simulink model "PTC_MBDS_HighpassT_RE_Sample"  (R2013a)
settings: Solver=FixedStepDiscrete  StartTime=0.0  StopTime=100  FixedStep=0.01  RelTol=1e-3
undefined symbols (not defined in the file): sigbuilder_block
libraries: simulink x2, simulink_extras x1, PTC_MBDS_LIB x1
settings Model: Creator=uidl7367  LastModifiedBy=sundeep.tuteja
settings DataIOCC: SignalLoggingSaveFormat=ModelDataLogs
settings OptimizationCC: ExpressionDepthLimit=2147483647  InitFltsAndDblsToZero=on
settings DebuggingCC: SaveWithParameterizedLinksMsg=none  SignalResolutionControl=TryResolveAllWithWarning  SolverPrmCheckMsg=none  InheritedTsInSrcMsg=none  MultiTaskDSMMsg=warning  MultiTaskCondExecSysMsg=none  FcnCallInpInsideContextMsg=UseLocalSettings  StrictBusMsg=Warning
settings RTWCC: IncludeERTFirstTime=on
settings GRTTargetCC: TargetFcnLib=ansi_tfl_tmw.mat  CombineOutputUpdateFcns=off  GRTInterface=on

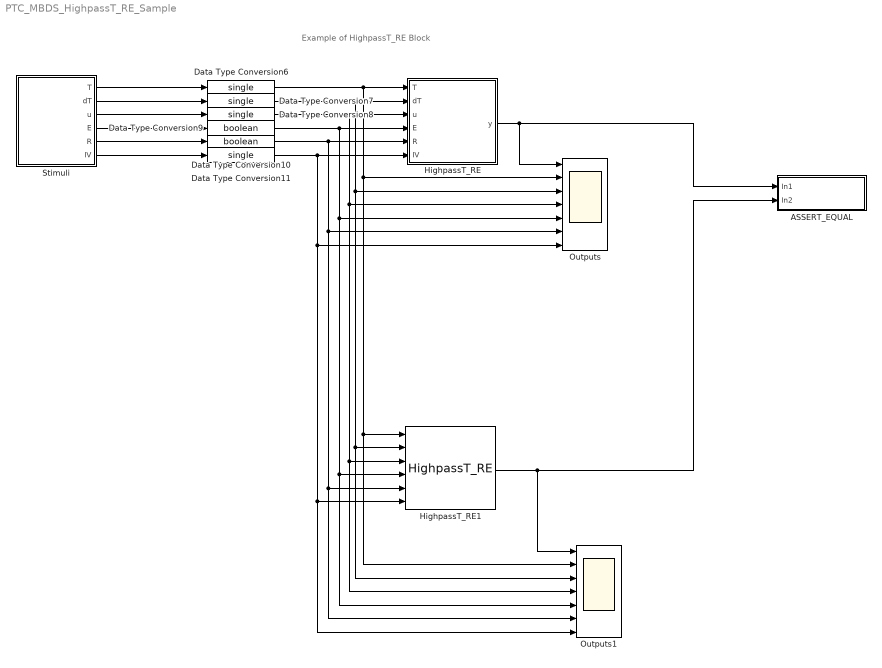
== system PTC_MBDS_HighpassT_RE_Sample ==
  note: Example of HighpassT_RE Block
  ASSERT_EQUAL : Subsystem
  Data Type Conversion10 : DataTypeConversion  InitFcn=|  OutDataTypeStr=boolean  SaturateOnIntegerOverflow=on
      | try
      |    MBDS_BlockCallback('Update', gcb);
      | end
  Data Type Conversion11 : DataTypeConversion  InitFcn=|  OutDataTypeStr=single  SaturateOnIntegerOverflow=on
      | try
      |    MBDS_BlockCallback('Update', gcb);
      | end
  Data Type Conversion6 : DataTypeConversion  InitFcn=|  OutDataTypeStr=single  SaturateOnIntegerOverflow=on
      | try
      |    MBDS_BlockCallback('Update', gcb);
      | end
  Data Type Conversion7 : DataTypeConversion  InitFcn=|  OutDataTypeStr=single  SaturateOnIntegerOverflow=on
      | try
      |    MBDS_BlockCallback('Update', gcb);
      | end
  Data Type Conversion8 : DataTypeConversion  InitFcn=|  OutDataTypeStr=single  SaturateOnIntegerOverflow=on
      | try
      |    MBDS_BlockCallback('Update', gcb);
      | end
  Data Type Conversion9 : DataTypeConversion  InitFcn=|  OutDataTypeStr=boolean  SaturateOnIntegerOverflow=on
      | try
      |    MBDS_BlockCallback('Update', gcb);
      | end
  HighpassT_RE : Subsystem  InitFcn=|  mask(HighpassT_RE){MBDS_LibraryBlock=on, dT_Enabled=on, dT=1, E_Enabled=on, R_Enabled=on, IV_Enabled=on, IV=0, MBDS_BlockVersion=05.40}
      | if(exist('MBDS_BlockCallback', 'file'))
      |    MBDS_BlockCallback('Update', gcb);
      | end
      mask prompts: MBDS_LibraryBlock "MBDS library block"; dT_Enabled "Show dT port"; dT "Sample rate (dT):"; E_Enabled "Show E port"; R_Enabled "Show R port"; IV_Enabled "Show IV port"; IV "Initial value (IV):"; MBDS_BlockVersion "Block version:"
      mask help: This block provides a discretized first order highpass filter with time constant T.
      mask init:
      | if(exist('MBDS_BlockCallback', 'file'))
      |    MBDS_BlockCallback('Init', gcb);
      | else
      |    % Disable all mask parameters
      |    MaskEnables = get_param(gcb, 'MaskEnables');
      |    for k = [1:length(MaskEnables)]
      |       MaskEnables{k} = 'off';
      |    end
      |    if(~isequal(MaskEnables, get_param(gcb, 'MaskEnables')))
      |       set_param(gcb, 'MaskEnables', MaskEnables);
      |    end
      | end
      mask Help: eval(['open([workdir(''library_dir:''),''\Blockset\help\'',get_param(gcb,''MaskType''),''.html''])'])
      mask Callback dT_Enabled:
      | % Update mask parameter dialog
      | if(exist('MBDS_BlockCallback', 'file'))
      |    MBDS_BlockCallback('dT_Enabled', gcb);
      | end
      mask Callback dT:
      | % Adopt Value
      | if(exist('MBDS_BlockCallback', 'file'))
      |    MBDS_BlockCallback('dT', gcb);
      | end
      mask Callback R_Enabled:
      | % Update mask parameter dialog
      | if(exist('MBDS_BlockCallback', 'file'))
      |    MBDS_BlockCallback('R_Enabled', gcb);
      | end
      mask Callback IV_Enabled:
      | % Update mask parameter dialog
      | if(exist('MBDS_BlockCallback', 'file'))
      |    MBDS_BlockCallback('IV_Enabled', gcb);
      | end
      mask Callback IV:
      | % Adopt Value
      | if(exist('MBDS_BlockCallback', 'file'))
      |    MBDS_BlockCallback('IV', gcb);
      | end
      mask Display:
      | % Show icon or block text
      | if(exist('HighpassT.tif', 'file'))
      |    image(imread('HighpassT.tif','tif'), [0.295739348370927 0.316666666666667 0.378947368421053 0.366666666666667]);
      |    disp('')
      | else
      |    disp(sprintf('Highpass'));
      | end
      | 
      | % Display port labels
      | port_label('input', 1, 'T');
      | port_label('input', 2, 'dT');
      | port_label('input', 3, 'u');
      | port_label('input', 4, 'E');
      | port_label('input', 5, 'R');
      | port_label('input', 6, 'IV');
      | port_label('output', 1, 'y');
  HighpassT_RE1 : PTC_MBDS_LIB/MBDS Standard Library/Extended Operations/Filters/HighpassT_RE  dT_Enabled=on  dT=1  E_Enabled=on  R_Enabled=on  IV_Enabled=on  IV=0  PTC_MBDS_BlockVersion=5.32  PTC_BlockType=PTC_MBDS_HighpassT_RE
  Outputs : Scope  NumInputPorts=7
      settings: TimeRange=10  YMin=-2~499~9~-2~-1~-1~0  YMax=2~501~11~2~1~1~2  SampleInput=on  SampleTime=0.01
  Outputs1 : Scope  NumInputPorts=7
      settings: TimeRange=10  YMin=-2~499~9~-2~-1~-1~0  YMax=2~501~11~2~1~1~2  SampleInput=on  SampleTime=0.01
  Stimuli : Subsystem  Tag=STV Subsys  LoadFcn=sigbuilder_block('load');  StartFcn=sigbuilder_block('start');  StopFcn=sigbuilder_block('stop');  ClipboardFcn=sigbuilder_block('clipboard');  mask(Sigbuilder block){}
      mask help: Sigbuilder GUI
      mask init:
      | if ~strcmp(get_param(bdroot(gcb),'SimulationStatus'),'stopped') tuvar = sigbuilder_block('maskInit'); end
      settings: CopyFcn=sigbuilder_block('copy');  DeleteFcn=sigbuilder_block('delete');  ModelCloseFcn=sigbuilder_block('modelClose');  PreSaveFcn=sigbuilder_block('preSave');  PauseFcn=sigbuilder_block('pause')  ContinueFcn=sigbuilder_block('continue')  NameChangeFcn=sigbuilder_block('namechange');  OpenFcn=sigbuilder_block('open',[207 70.5 730.5 612 ]);  CloseFcn=sigbuilder_block('close');
      mask Display: plot(0,0,100,100,[10,10,40,40,10],[80,20,20,80,80],[40,10],[50,50], [40,27,10],[65,72,56],[40,25,25,10],[28,28,43,43]);
  wires:
  Stimuli/2(dT) -> Data Type Conversion7/1
  Stimuli/1(T) -> Data Type Conversion6/1
  Stimuli/3(u) -> Data Type Conversion8/1
  Stimuli/4(E) -> Data Type Conversion9/1
  Stimuli/5(R) -> Data Type Conversion10/1
  Stimuli/6(IV) -> Data Type Conversion11/1
  Data Type Conversion7/1 -> HighpassT_RE/2(dT), HighpassT_RE1/2, Outputs1/3, Outputs/3
  Data Type Conversion9/1 -> HighpassT_RE/4(E), HighpassT_RE1/4, Outputs1/5, Outputs/5
  Data Type Conversion8/1 -> HighpassT_RE/3(u), HighpassT_RE1/3, Outputs1/4, Outputs/4
  Data Type Conversion10/1 -> HighpassT_RE/5(R), HighpassT_RE1/5, Outputs1/6, Outputs/6
  Data Type Conversion6/1 -> HighpassT_RE/1(T), HighpassT_RE1/1, Outputs1/2, Outputs/2
  Data Type Conversion11/1 -> HighpassT_RE/6(IV), Outputs/7, HighpassT_RE1/6, Outputs1/7
  HighpassT_RE/1(y) -> ASSERT_EQUAL/1(In1), Outputs/1
  HighpassT_RE1/1 -> ASSERT_EQUAL/2(In2), Outputs1/1

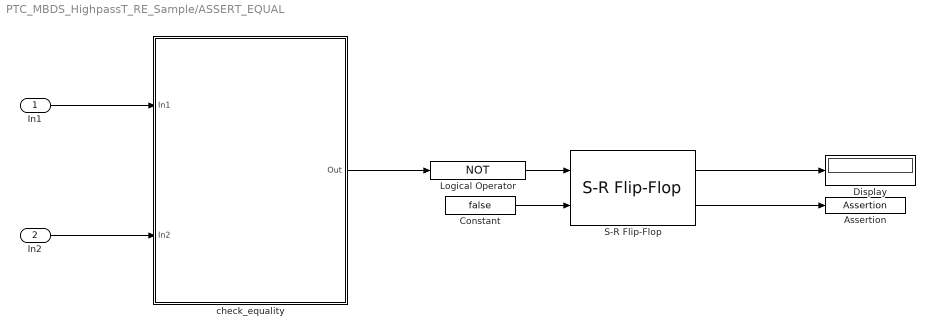
== system PTC_MBDS_HighpassT_RE_Sample/ASSERT_EQUAL ==
  In1 : Inport
  In2 : Inport  Port=2
  Assertion : Assertion
  Constant : Constant  Value=false
  Display : Display
  Logical Operator : Logic  Operator=NOT  AllPortsSameDT=off  OutDataTypeStr=boolean
  S-R Flip-Flop : simulink_extras/Flip Flops/S-R Flip-Flop  initial_condition=0
  check_equality : MATLAB Function  TreatAsAtomicUnit=on
  wires:
  S-R Flip-Flop/1 -> Display/1
  check_equality/1(Out) -> Logical Operator/1
  Constant/1 -> S-R Flip-Flop/2
  S-R Flip-Flop/2 -> Assertion/1
  In2/1 -> check_equality/2(In2)
  In1/1 -> check_equality/1(In1)
  Logical Operator/1 -> S-R Flip-Flop/1

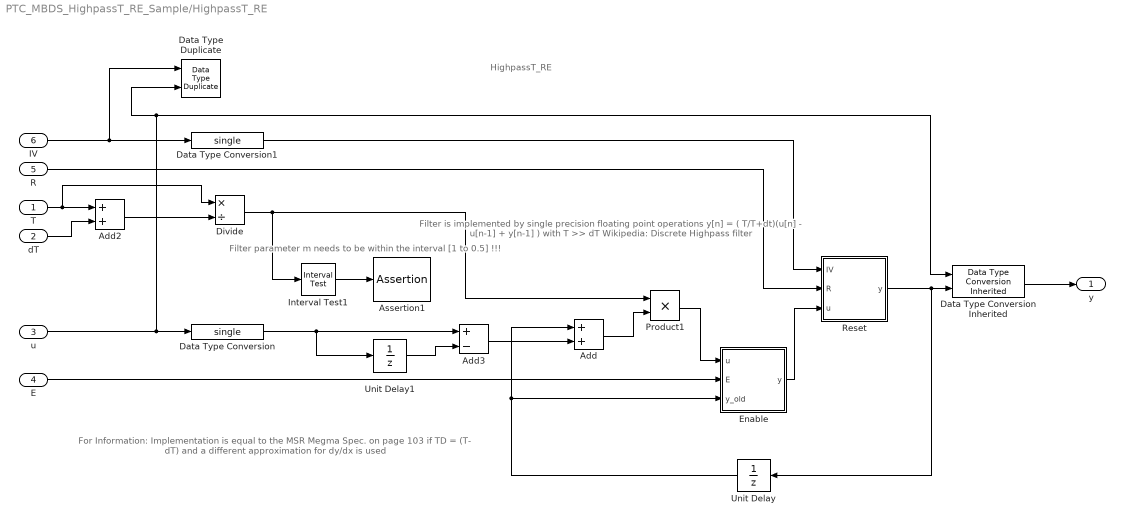
== system PTC_MBDS_HighpassT_RE_Sample/HighpassT_RE ==
  note: For Information:
      | Implementation is equal to the MSR Megma Spec. on page 103 if
      | TD = (T- dT) and a different approximation for dy/dx is used
  note: HighpassT_RE
  note: Filter is implemented by single
      | precision floating point operations
      |
      | y[n] = ( T/T+dt)(u[n] - u[n-1] + y[n-1] )
      | with T >> dT
      |
      | Wikipedia: Discrete Highpass filter
  note: Filter parameter m needs to
      | be within the interval [1 to 0.5] !!!
  T : Inport
  dT : Inport  Port=2
  u : Inport  Port=3
  E : Inport  Port=4  OutDataTypeStr=boolean
  R : Inport  Port=5  OutDataTypeStr=boolean
  IV : Inport  Port=6
  Add : Sum  OutDataTypeStr=Inherit: Inherit via back propagation
  Add2 : Sum  OutDataTypeStr=Inherit: Inherit via back propagation
  Add3 : Sum  Inputs=+-  OutDataTypeStr=Inherit: Inherit via back propagation
  Assertion1 : Assertion  AssertionFailFcn="error('Filter parameter m has to be within the interval  of [0..1]. ')"
  Data Type Conversion Inherited : simulink/Signal Attributes/Data Type Conversion Inherited  ConvertRealWorld=Real World Value  RndMeth=Nearest  DoSatur=off
  Data Type Duplicate : DataTypeDuplicate
  Data Type Conversion : DataTypeConversion  OutDataTypeStr=single
  Data Type Conversion1 : DataTypeConversion  OutDataTypeStr=single
  Divide : Product  Inputs=*/  OutDataTypeStr=single
  Enable : Subsystem
  Interval Test1 : simulink/Logic and Bit Operations/Interval Test  IntervalClosedRight=on  uplimit=1  IntervalClosedLeft=on  lowlimit=0.5  OutDataTypeStr=boolean
  Product1 : Product  OutDataTypeStr=Inherit: Inherit via back propagation  RndMeth=Zero
  Reset : Subsystem
  Unit Delay : UnitDelay  SampleTime=-1
  Unit Delay1 : UnitDelay  SampleTime=-1
  y : Outport
  wires:
  Unit Delay1/1 -> Add3/2
  Unit Delay/1 -> Add/1, Enable/3(y_old)
  Add3/1 -> Add/2
  Data Type Conversion/1 -> Unit Delay1/1, Add3/1
  Reset/1(y) -> Unit Delay/1, Data Type Conversion Inherited/2
  Enable/1(y) -> Reset/3(u)
  R/1 -> Reset/2(R)
  Data Type Conversion1/1 -> Reset/1(IV)
  E/1 -> Enable/2(E)
  Add/1 -> Product1/2
  Data Type Conversion Inherited/1 -> y/1
  u/1 -> Data Type Duplicate/2, Data Type Conversion Inherited/1, Data Type Conversion/1
  IV/1 -> Data Type Conversion1/1, Data Type Duplicate/1
  T/1 -> Add2/1, Divide/1
  dT/1 -> Add2/2
  Add2/1 -> Divide/2
  Product1/1 -> Enable/1(u)
  Interval Test1/1 -> Assertion1/1
  Divide/1 -> Interval Test1/1, Product1/1

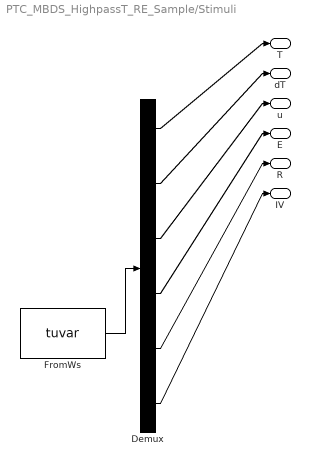
== system PTC_MBDS_HighpassT_RE_Sample/Stimuli ==
  Demux : Demux  Tag=STV Demux  Outputs=6
  FromWs : FromWorkspace  Tag=STV FromWs  VariableName=tuvar  SampleTime=0  OutputAfterFinalValue=Holding final value
      SigBuilderData=|
      | common.afterFinalStr = 'Hold final value'
      | common.sampleTime = 0
      | dataSet.timeRange = [0 10]
      | dataSet.name = 'test data'
      | sbobj.Groups.Name = 'test data'
      | sbobj.Groups.Signals(1).Name = 'T'
      | sbobj.Groups.Signals(1).XData = [0 10]
      | sbobj.Groups.Signals(1).YData = [500 500]
      | sbobj.Groups.Signals(2).Name = 'dT'
      | sbobj.Groups.Signals(2).XData = [0 10]
      | sbobj.Groups.Signals(2).YData = [10 10]
      | sbobj.Groups.Signals(3).Name = 'u'
      | sbobj.Groups.Signals(3).XData = [0 6 6 10]
      | sbobj.Groups.Signals(3).YData = [0 0 0.98 0.98]
      | sbobj.Groups.Signals(4).Name = 'E'
      | sbobj.Groups.Signals(4).XData = [0 8 8 10]
      | sbobj.Groups.Signals(4).YData = [1 1 0 0]
      | sbobj.Groups.Signals(5).Name = 'R'
      | sbobj.Groups.Signals(5).XData = [0 1.02 1.02 1.24 1.24 10]
      | sbobj.Groups.Signals(5).YData = [0 0 1 1 0 0]
      | sbobj.Groups.Signals(6).Name = 'IV'
      | sbobj.Groups.Signals(6).XData = [0 10]
      | sbobj.Groups.Signals(6).YData = [0.5 0.5]
  T : Outport  Tag=STV Outport
  dT : Outport  Tag=STV Outport  Port=2
  u : Outport  Tag=STV Outport  Port=3
  E : Outport  Tag=STV Outport  Port=4
  R : Outport  Tag=STV Outport  Port=5
  IV : Outport  Tag=STV Outport  Port=6
  wires:
  Demux/6 -> IV/1
  Demux/5 -> R/1
  Demux/4 -> E/1
  Demux/3 -> u/1
  Demux/2 -> dT/1
  Demux/1 -> T/1
  FromWs/1 -> Demux/1

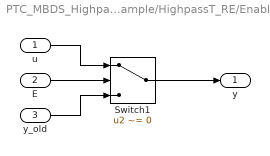
== system PTC_MBDS_HighpassT_RE_Sample/HighpassT_RE/Enable ==
  u : Inport
  E : Inport  Port=2
  y_old : Inport  Port=3
  Switch1 : Switch  Criteria=u2 ~= 0  OutDataTypeStr=Inherit: Inherit via back propagation  InputSameDT=on
  y : Outport
  wires:
  y_old/1 -> Switch1/3
  Switch1/1 -> y/1
  u/1 -> Switch1/1
  E/1 -> Switch1/2

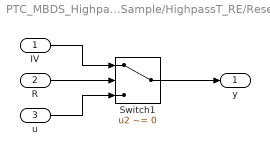
== system PTC_MBDS_HighpassT_RE_Sample/HighpassT_RE/Reset ==
  IV : Inport
  R : Inport  Port=2
  u : Inport  Port=3
  Switch1 : Switch  Criteria=u2 ~= 0  OutDataTypeStr=Inherit: Inherit via back propagation  InputSameDT=on
  y : Outport
  wires:
  u/1 -> Switch1/3
  Switch1/1 -> y/1
  IV/1 -> Switch1/1
  R/1 -> Switch1/2

== matlab function PTC_MBDS_HighpassT_RE_Sample/ASSERT_EQUAL/check_equality ==
  data: In1 input; Out output; In2 input
function Out = check_equality(In1, In2)
%#codegen

Out = isequaln(In1, In2);

end
